simulink library "Computer_Library"  (Simulink 8.1)
settings: Solver=ode45  StartTime=0.0  StopTime=10.0  RelTol=1e-3
values from neighbouring files (symbols this model uses):
  A = 10    [CharTable.m]
  ARROW_DOWN = 48    [CharTable.m]
  ARROW_LEFT = 49    [CharTable.m]
  ARROW_RIGHT = 50    [CharTable.m]
  ARROW_UP = 47    [CharTable.m]
  ASTERISK = 39    [CharTable.m]
  B = 11    [CharTable.m]
  BACKSLASH = 43    [CharTable.m]
  C = 12    [CharTable.m]
  COLON = 40    [CharTable.m]
  COMMA = 53    [CharTable.m]
  CROSS = 38    [CharTable.m]
  CURSOR = 62    [CharTable.m]
  D = 13    [CharTable.m]
  DOT = 52    [CharTable.m]
  EQUAL = 44    [CharTable.m]
  EXCLAMATION_MARK = 55    [CharTable.m]
  F = 15    [CharTable.m]
  G = 16    [CharTable.m]
  GREATER_THAN = 46    [CharTable.m]
  H = 17    [CharTable.m]
  I = 18    [CharTable.m]
  J = 19    [CharTable.m]
  K = 20    [CharTable.m]
  L = 21    [CharTable.m]
  LEFT_PARENTHESES = 59    [CharTable.m]
  LESS_THAN = 45    [CharTable.m]
  M = 22    [CharTable.m]
  MINUS = 37    [CharTable.m]
  N = 23    [CharTable.m]
  O = 24    [CharTable.m]
  P = 25    [CharTable.m]
  PERCENT = 58    [CharTable.m]
  PLUS = 36    [CharTable.m]
  Q = 32    [CharTable.m]
  QUESTION_MARK = 54    [CharTable.m]
  QUOTE = 56    [CharTable.m]
  R = 26    [CharTable.m]
  RECTANGLE = 63    [CharTable.m]
  RIGHT_PARENTHESES = 60    [CharTable.m]
  RomCode = reshape(transpose(RomCode), [], 1)    [ROM.m]
  S = 27    [CharTable.m]
  SEMICOLON = 41    [CharTable.m]
  SHARP = 57    [CharTable.m]
  SLASH = 42    [CharTable.m]
  SPACE = 61    [CharTable.m]
  T = 28    [CharTable.m]
  U = 29    [CharTable.m]
  UNDERSCORE = 51    [CharTable.m]
  V = 30    [CharTable.m]
  W = 31    [CharTable.m]
  X = 33    [CharTable.m]
  Y = 34    [CharTable.m]
  Z = 35    [CharTable.m]
undefined symbols (not defined in the file or in its folder): char_0
libraries: Memory_Blocks_Lib x116, Byte_Multiplexers_Lib x44, commutil2 x18, Bit_Multiplexers_Lib x17, Decoders_Lib x9, simulink_extras x8, Logic_Operations_Lib x4, Byte_Demultiplexers_Lib x2, Arithmetic_Operations_Lib x2, dspsnks4 x1
(part 1 of 4)
settings Model: Creator=N  LastModifiedBy=uzivatel

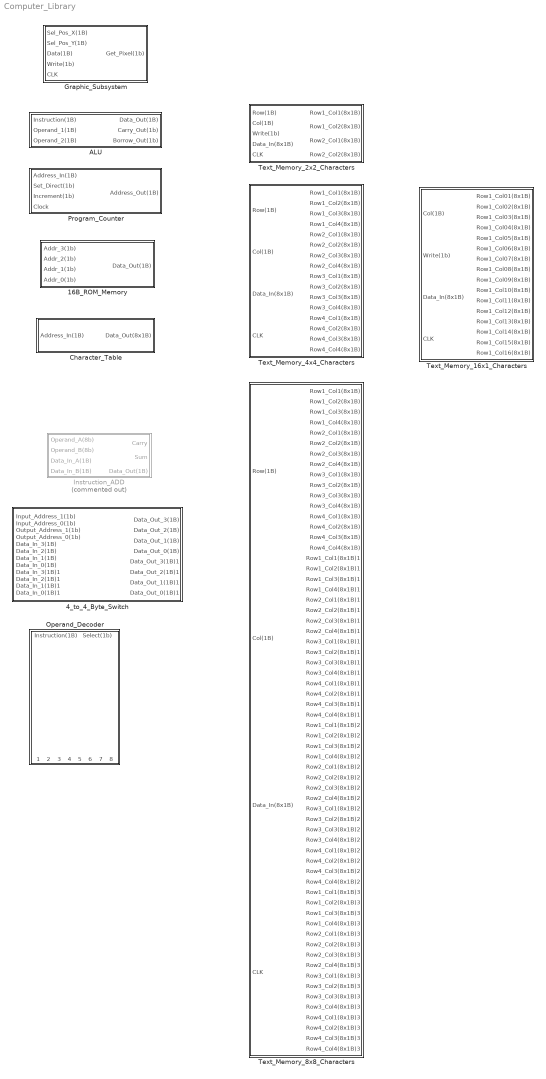
== system Computer_Library ==
  16B_ROM_Memory : Subsystem
  4_to_4_Byte_Switch : Subsystem
  ALU : Subsystem
  Character_Table : Subsystem
  Graphic_Subsystem : Subsystem
  Instruction_ADD : Subsystem  Commented=on
  Operand_Decoder : Subsystem
  Program_Counter : Subsystem
  Text_Memory_16x1_Characters : Subsystem
  Text_Memory_2x2_Characters : Subsystem
  Text_Memory_4x4_Characters : Subsystem
  Text_Memory_8x8_Characters : Subsystem

== system Computer_Library/16B_ROM_Memory ==
  Addr_3(1b) : Inport
  Addr_2(1b) : Inport  Port=2
  Addr_1(1b) : Inport  Port=3
  Addr_0(1b) : Inport  Port=4
  16_to_1_Byte_Multiplexer : Byte_Multiplexers_Lib/Byte_Multiplexers_Lib/Byte_Multiplexer_16_to_1
  Byte_00 : Constant  Value=RomCode(1)  OutDataTypeStr=uint8
  Byte_01 : Constant  Value=RomCode(2)  OutDataTypeStr=uint8
  Byte_02 : Constant  Value=RomCode(3)  OutDataTypeStr=uint8
  Byte_03 : Constant  Value=RomCode(4)  OutDataTypeStr=uint8
  Byte_04 : Constant  Value=RomCode(5)  OutDataTypeStr=uint8
  Byte_05 : Constant  Value=RomCode(6)  OutDataTypeStr=uint8
  Byte_06 : Constant  Value=RomCode(7)  OutDataTypeStr=uint8
  Byte_07 : Constant  Value=RomCode(8)  OutDataTypeStr=uint8
  Byte_08 : Constant  Value=RomCode(9)  OutDataTypeStr=uint8
  Byte_09 : Constant  Value=RomCode(10)  OutDataTypeStr=uint8
  Byte_10 : Constant  Value=RomCode(11)  OutDataTypeStr=uint8
  Byte_11 : Constant  Value=RomCode(12)  OutDataTypeStr=uint8
  Byte_12 : Constant  Value=RomCode(13)  OutDataTypeStr=uint8
  Byte_13 : Constant  Value=RomCode(14)  OutDataTypeStr=uint8
  Byte_14 : Constant  Value=RomCode(15)  OutDataTypeStr=uint8
  Byte_15 : Constant  Value=RomCode(16)  OutDataTypeStr=uint8
  Data_Out(1B) : Outport
  wires:
  16_to_1_Byte_Multiplexer/1 -> Data_Out(1B)/1
  Byte_00/1 -> 16_to_1_Byte_Multiplexer/20
  Byte_01/1 -> 16_to_1_Byte_Multiplexer/19
  Byte_02/1 -> 16_to_1_Byte_Multiplexer/18
  Byte_03/1 -> 16_to_1_Byte_Multiplexer/17
  Byte_04/1 -> 16_to_1_Byte_Multiplexer/16
  Byte_05/1 -> 16_to_1_Byte_Multiplexer/15
  Byte_06/1 -> 16_to_1_Byte_Multiplexer/14
  Byte_07/1 -> 16_to_1_Byte_Multiplexer/13
  Byte_08/1 -> 16_to_1_Byte_Multiplexer/12
  Byte_09/1 -> 16_to_1_Byte_Multiplexer/11
  Byte_10/1 -> 16_to_1_Byte_Multiplexer/10
  Byte_11/1 -> 16_to_1_Byte_Multiplexer/9
  Byte_12/1 -> 16_to_1_Byte_Multiplexer/8
  Byte_13/1 -> 16_to_1_Byte_Multiplexer/7
  Byte_14/1 -> 16_to_1_Byte_Multiplexer/6
  Byte_15/1 -> 16_to_1_Byte_Multiplexer/5
  Addr_3(1b)/1 -> 16_to_1_Byte_Multiplexer/1
  Addr_2(1b)/1 -> 16_to_1_Byte_Multiplexer/2
  Addr_1(1b)/1 -> 16_to_1_Byte_Multiplexer/3
  Addr_0(1b)/1 -> 16_to_1_Byte_Multiplexer/4

== system Computer_Library/4_to_4_Byte_Switch ==
  Input_Address_1(1b) : Inport
  Input_Address_0(1b) : Inport  Port=2
  Output_Address_1(1b) : Inport  Port=3
  Output_Address_0(1b) : Inport  Port=4
  Data_In_3(1B) : Inport  Port=5
  Data_In_2(1B) : Inport  Port=6
  Data_In_1(1B) : Inport  Port=7
  Data_In_0(1B) : Inport  Port=8
  Data_In_3(1B)1 : Inport  Port=9
  Data_In_2(1B)1 : Inport  Port=10
  Data_In_1(1B)1 : Inport  Port=11
  Data_In_0(1B)1 : Inport  Port=12
  1_to_4_Byte_Demultiplexer : Byte_Demultiplexers_Lib/Byte_Demultiplexers_Lib/Byte_Demultiplexer_1_to_4
  1_to_4_Byte_Demultiplexer1 : Byte_Demultiplexers_Lib/Byte_Demultiplexers_Lib/Byte_Demultiplexer_1_to_4
  4_to_1_Byte_Multiplexer1 : Byte_Multiplexers_Lib/Byte_Multiplexers_Lib/Byte_Multiplexer_4_to_1
  4_to_1_Byte_Multiplexer4 : Byte_Multiplexers_Lib/Byte_Multiplexers_Lib/Byte_Multiplexer_4_to_1
  Data_Out_3(1B) : Outport
  Data_Out_2(1B) : Outport  Port=2
  Data_Out_1(1B) : Outport  Port=3
  Data_Out_0(1B) : Outport  Port=4
  Data_Out_3(1B)1 : Outport  Port=5
  Data_Out_2(1B)1 : Outport  Port=6
  Data_Out_1(1B)1 : Outport  Port=7
  Data_Out_0(1B)1 : Outport  Port=8
  wires:
  4_to_1_Byte_Multiplexer4/1 -> 1_to_4_Byte_Demultiplexer/3
  1_to_4_Byte_Demultiplexer/1 -> Data_Out_3(1B)/1
  1_to_4_Byte_Demultiplexer/2 -> Data_Out_2(1B)/1
  1_to_4_Byte_Demultiplexer/3 -> Data_Out_1(1B)/1
  1_to_4_Byte_Demultiplexer/4 -> Data_Out_0(1B)/1
  Data_In_0(1B)/1 -> 4_to_1_Byte_Multiplexer4/6
  Data_In_1(1B)/1 -> 4_to_1_Byte_Multiplexer4/5
  Data_In_2(1B)/1 -> 4_to_1_Byte_Multiplexer4/4
  Data_In_3(1B)/1 -> 4_to_1_Byte_Multiplexer4/3
  Input_Address_0(1b)/1 -> 1_to_4_Byte_Demultiplexer1/2, 4_to_1_Byte_Multiplexer4/2
  Input_Address_1(1b)/1 -> 1_to_4_Byte_Demultiplexer1/1, 4_to_1_Byte_Multiplexer4/1
  Output_Address_0(1b)/1 -> 4_to_1_Byte_Multiplexer1/2, 1_to_4_Byte_Demultiplexer/2
  Output_Address_1(1b)/1 -> 4_to_1_Byte_Multiplexer1/1, 1_to_4_Byte_Demultiplexer/1
  4_to_1_Byte_Multiplexer1/1 -> 1_to_4_Byte_Demultiplexer1/3
  1_to_4_Byte_Demultiplexer1/1 -> Data_Out_3(1B)1/1
  1_to_4_Byte_Demultiplexer1/2 -> Data_Out_2(1B)1/1
  1_to_4_Byte_Demultiplexer1/3 -> Data_Out_1(1B)1/1
  1_to_4_Byte_Demultiplexer1/4 -> Data_Out_0(1B)1/1
  Data_In_0(1B)1/1 -> 4_to_1_Byte_Multiplexer1/6
  Data_In_1(1B)1/1 -> 4_to_1_Byte_Multiplexer1/5
  Data_In_2(1B)1/1 -> 4_to_1_Byte_Multiplexer1/4
  Data_In_3(1B)1/1 -> 4_to_1_Byte_Multiplexer1/3

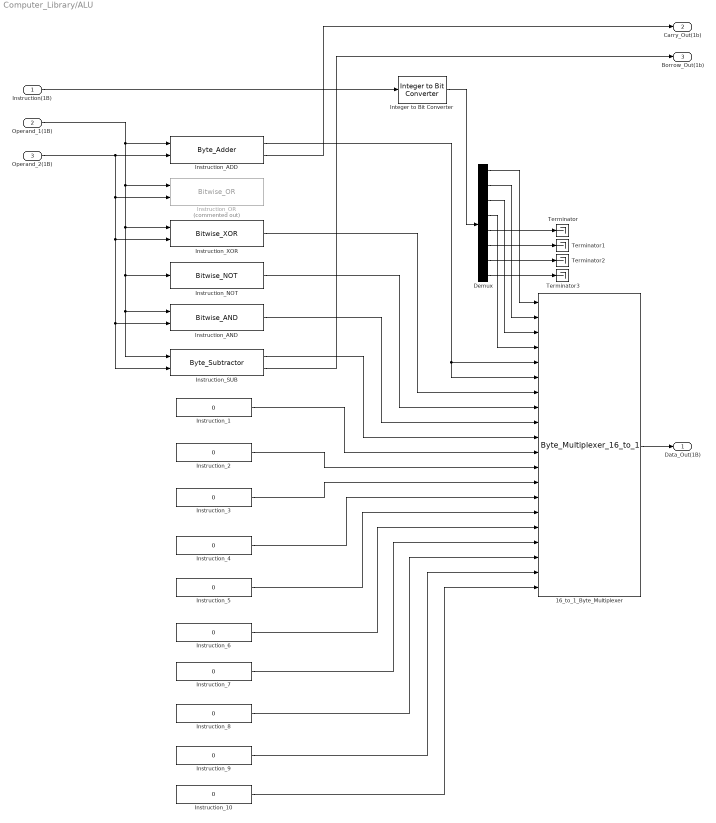
== system Computer_Library/ALU ==
  Instruction(1B) : Inport
  Operand_1(1B) : Inport  Port=2
  Operand_2(1B) : Inport  Port=3
  16_to_1_Byte_Multiplexer : Byte_Multiplexers_Lib/Byte_Multiplexers_Lib/Byte_Multiplexer_16_to_1
  Demux : Demux  Outputs=8
  Instruction_{1..10} (10 alike) : Constant  Value=0  OutDataTypeStr=uint8
  Instruction_ADD : Arithmetic_Operations_Lib/Arithmetic_Operations_Lib/Byte_Adder
  Instruction_AND : Logic_Operations_Lib/Logic_Operations_Lib/Bitwise_AND
  Instruction_NOT : Logic_Operations_Lib/Logic_Operations_Lib/Bitwise_NOT
  Instruction_OR : Logic_Operations_Lib/Logic_Operations_Lib/Bitwise_OR  Commented=on
  Instruction_SUB : Arithmetic_Operations_Lib/Arithmetic_Operations_Lib/Byte_Subtractor
  Instruction_XOR : Logic_Operations_Lib/Logic_Operations_Lib/Bitwise_XOR
  Integer to Bit Converter : commutil2/Integer to Bit Converter  nbits=8  signedInputValues=Unsigned  bitOrder=MSB first  outDtype=boolean
  Terminator{,1..3} (4 alike) : Terminator
  Data_Out(1B) : Outport
  Carry_Out(1b) : Outport  Port=2
  Borrow_Out(1b) : Outport  Port=3
  wires:
  Operand_1(1B)/1 -> Instruction_OR/1, Instruction_AND/1, Instruction_SUB/1, Instruction_NOT/1, Instruction_XOR/1, Instruction_ADD/1
  Operand_2(1B)/1 -> Instruction_OR/2, Instruction_AND/2, Instruction_SUB/2, Instruction_XOR/2, Instruction_ADD/2
  Instruction_ADD/1 -> 16_to_1_Byte_Multiplexer/6, 16_to_1_Byte_Multiplexer/5
  Instruction_XOR/1 -> 16_to_1_Byte_Multiplexer/7
  Instruction_NOT/1 -> 16_to_1_Byte_Multiplexer/8
  Instruction_AND/1 -> 16_to_1_Byte_Multiplexer/9
  Instruction_SUB/1 -> 16_to_1_Byte_Multiplexer/10
  Instruction_1/1 -> 16_to_1_Byte_Multiplexer/11
  Instruction_2/1 -> 16_to_1_Byte_Multiplexer/12
  Instruction_3/1 -> 16_to_1_Byte_Multiplexer/13
  Instruction_4/1 -> 16_to_1_Byte_Multiplexer/14
  Instruction_5/1 -> 16_to_1_Byte_Multiplexer/15
  Instruction_6/1 -> 16_to_1_Byte_Multiplexer/16
  Instruction_7/1 -> 16_to_1_Byte_Multiplexer/17
  Instruction_8/1 -> 16_to_1_Byte_Multiplexer/18
  Instruction_9/1 -> 16_to_1_Byte_Multiplexer/19
  Instruction_10/1 -> 16_to_1_Byte_Multiplexer/20
  Instruction(1B)/1 -> Integer to Bit Converter/1
  16_to_1_Byte_Multiplexer/1 -> Data_Out(1B)/1
  Integer to Bit Converter/1 -> Demux/1
  Demux/4 -> 16_to_1_Byte_Multiplexer/4
  Demux/3 -> 16_to_1_Byte_Multiplexer/3
  Demux/2 -> 16_to_1_Byte_Multiplexer/2
  Demux/1 -> 16_to_1_Byte_Multiplexer/1
  Demux/8 -> Terminator3/1
  Demux/7 -> Terminator2/1
  Demux/6 -> Terminator1/1
  Demux/5 -> Terminator/1
  Instruction_ADD/2 -> Carry_Out(1b)/1
  Instruction_SUB/2 -> Borrow_Out(1b)/1

== system Computer_Library/Character_Table ==
  note: Toto nie su stlpce ale riadky, treba opravit!!!
  Address_In(1B) : Inport
  4_to_1_Byte_Multiplexer{,1..7} (8 alike) : Byte_Multiplexers_Lib/Byte_Multiplexers_Lib/Byte_Multiplexer_4_to_1
  Characters(0..F) : Subsystem
  Characters(ARROW_DOWN..RECTANGLE) : Subsystem
  Characters(G..W) : Subsystem
  Characters(Q..ARROW_UP) : Subsystem
  Demux : Demux  Outputs=8
  Integer to Bit Converter : commutil2/Integer to Bit Converter  nbits=8  signedInputValues=Unsigned  bitOrder=MSB first  outDtype=uint8
  Mux : Mux  Inputs=8
  Terminator : Terminator
  Terminator1 : Terminator
  Data_Out(8x1B) : Outport
  wires:
  Characters(0..F)/3(Column_3(1B)) -> 4_to_1_Byte_Multiplexer2/6
  Characters(Q..ARROW_UP)/6(Column_6(1B)) -> 4_to_1_Byte_Multiplexer5/4
  Characters(Q..ARROW_UP)/7(Column_7(1B)) -> 4_to_1_Byte_Multiplexer6/4
  Characters(ARROW_DOWN..RECTANGLE)/2(Column_2(1B)) -> 4_to_1_Byte_Multiplexer1/3
  Characters(0..F)/2(Column_2(1B)) -> 4_to_1_Byte_Multiplexer1/6
  Characters(Q..ARROW_UP)/2(Column_2(1B)) -> 4_to_1_Byte_Multiplexer1/4
  Characters(ARROW_DOWN..RECTANGLE)/7(Column_7(1B)) -> 4_to_1_Byte_Multiplexer6/3
  Characters(G..W)/2(Column_2(1B)) -> 4_to_1_Byte_Multiplexer1/5
  Characters(ARROW_DOWN..RECTANGLE)/8(Column_8(1B)) -> 4_to_1_Byte_Multiplexer7/3
  Characters(G..W)/4(Column_4(1B)) -> 4_to_1_Byte_Multiplexer3/5
  Characters(ARROW_DOWN..RECTANGLE)/6(Column_6(1B)) -> 4_to_1_Byte_Multiplexer5/3
  Characters(G..W)/3(Column_3(1B)) -> 4_to_1_Byte_Multiplexer2/5
  Characters(Q..ARROW_UP)/5(Column_5(1B)) -> 4_to_1_Byte_Multiplexer4/4
  Characters(0..F)/4(Column_4(1B)) -> 4_to_1_Byte_Multiplexer3/6
  Characters(Q..ARROW_UP)/1(Column_1(1B)) -> 4_to_1_Byte_Multiplexer/4
  Characters(ARROW_DOWN..RECTANGLE)/3(Column_3(1B)) -> 4_to_1_Byte_Multiplexer2/3
  Characters(Q..ARROW_UP)/3(Column_3(1B)) -> 4_to_1_Byte_Multiplexer2/4
  Characters(G..W)/6(Column_6(1B)) -> 4_to_1_Byte_Multiplexer5/5
  Characters(0..F)/7(Column_7(1B)) -> 4_to_1_Byte_Multiplexer6/6
  Characters(G..W)/7(Column_7(1B)) -> 4_to_1_Byte_Multiplexer6/5
  Characters(0..F)/8(Column_8(1B)) -> 4_to_1_Byte_Multiplexer7/6
  Characters(Q..ARROW_UP)/8(Column_8(1B)) -> 4_to_1_Byte_Multiplexer7/4
  Characters(ARROW_DOWN..RECTANGLE)/5(Column_5(1B)) -> 4_to_1_Byte_Multiplexer4/3
  Characters(G..W)/8(Column_8(1B)) -> 4_to_1_Byte_Multiplexer7/5
  Demux/3 -> 4_to_1_Byte_Multiplexer1/1, 4_to_1_Byte_Multiplexer2/1, 4_to_1_Byte_Multiplexer4/1, 4_to_1_Byte_Multiplexer5/1, 4_to_1_Byte_Multiplexer6/1, 4_to_1_Byte_Multiplexer7/1, 4_to_1_Byte_Multiplexer3/1, 4_to_1_Byte_Multiplexer/1
  Characters(Q..ARROW_UP)/4(Column_4(1B)) -> 4_to_1_Byte_Multiplexer3/4
  Demux/4 -> 4_to_1_Byte_Multiplexer1/2, 4_to_1_Byte_Multiplexer2/2, 4_to_1_Byte_Multiplexer3/2, 4_to_1_Byte_Multiplexer4/2, 4_to_1_Byte_Multiplexer5/2, 4_to_1_Byte_Multiplexer6/2, 4_to_1_Byte_Multiplexer7/2, 4_to_1_Byte_Multiplexer/2
  Characters(0..F)/1(Column_1(1B)) -> 4_to_1_Byte_Multiplexer/6
  Characters(G..W)/1(Column_1(1B)) -> 4_to_1_Byte_Multiplexer/5
  Characters(0..F)/5(Column_5(1B)) -> 4_to_1_Byte_Multiplexer4/6
  Characters(G..W)/5(Column_5(1B)) -> 4_to_1_Byte_Multiplexer4/5
  Characters(0..F)/6(Column_6(1B)) -> 4_to_1_Byte_Multiplexer5/6
  Characters(ARROW_DOWN..RECTANGLE)/1(Column_1(1B)) -> 4_to_1_Byte_Multiplexer/3
  Characters(ARROW_DOWN..RECTANGLE)/4(Column_4(1B)) -> 4_to_1_Byte_Multiplexer3/3
  Demux/8 -> Characters(ARROW_DOWN..RECTANGLE)/4(Address_0_In(1b)), Characters(Q..ARROW_UP)/4(Address_0_In(1b)), Characters(G..W)/4(Address_0_In(1b)), Characters(0..F)/4(Address_0_In(1b))
  Demux/6 -> Characters(ARROW_DOWN..RECTANGLE)/2(Address_2_In(1b)), Characters(Q..ARROW_UP)/2(Address_2_In(1b)), Characters(0..F)/2(Address_2_In(1b)), Characters(G..W)/2(Address_2_In(1b))
  4_to_1_Byte_Multiplexer6/1 -> Mux/7
  Demux/5 -> Characters(ARROW_DOWN..RECTANGLE)/1(Address_3_In(1b)), Characters(Q..ARROW_UP)/1(Address_3_In(1b)), Characters(G..W)/1(Address_3_In(1b)), Characters(0..F)/1(Address_3_In(1b))
  4_to_1_Byte_Multiplexer1/1 -> Mux/2
  4_to_1_Byte_Multiplexer5/1 -> Mux/6
  4_to_1_Byte_Multiplexer2/1 -> Mux/3
  4_to_1_Byte_Multiplexer3/1 -> Mux/4
  4_to_1_Byte_Multiplexer7/1 -> Mux/8
  4_to_1_Byte_Multiplexer/1 -> Mux/1
  Demux/7 -> Characters(ARROW_DOWN..RECTANGLE)/3(Address_1_In(1b)), Characters(Q..ARROW_UP)/3(Address_1_In(1b)), Characters(0..F)/3(Address_1_In(1b)), Characters(G..W)/3(Address_1_In(1b))
  4_to_1_Byte_Multiplexer4/1 -> Mux/5
  Address_In(1B)/1 -> Integer to Bit Converter/1
  Demux/1 -> Terminator/1
  Demux/2 -> Terminator1/1
  Integer to Bit Converter/1 -> Demux/1
  Mux/1 -> Data_Out(8x1B)/1

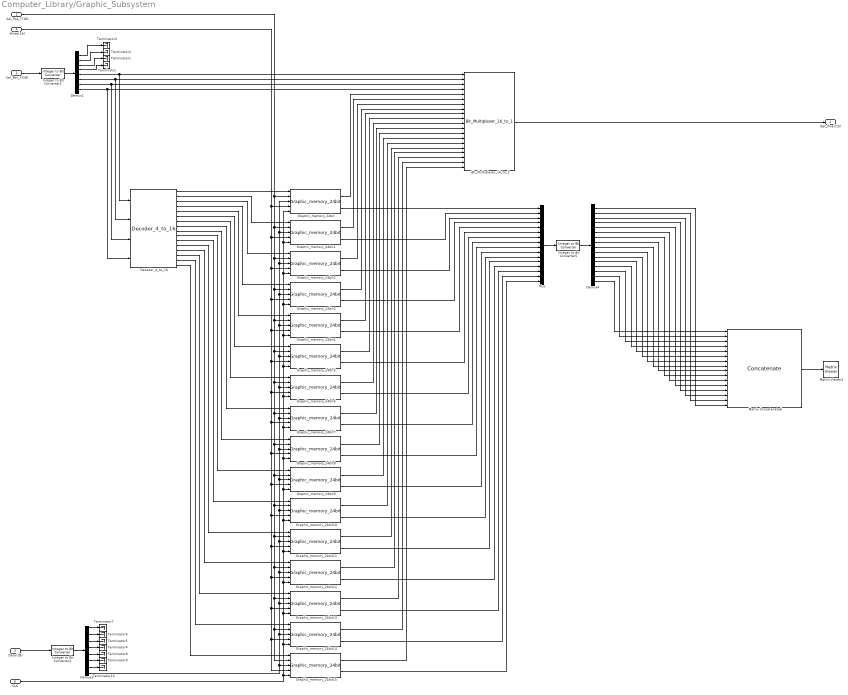
== system Computer_Library/Graphic_Subsystem ==
  Sel_Pos_X(1B) : Inport
  Sel_Pos_Y(1B) : Inport  Port=2
  Data(1B) : Inport  Port=3
  Write(1b) : Inport  Port=4
  CLK : Inport  Port=5
  Bit_Multiplexer_16_to_1 : Bit_Multiplexers_Lib/Bit_Multiplexers_Lib/Bit_Multiplexer_16_to_1
  Decoder_4_to_16 : Decoders_Lib/Decoders_Lib/Decoder_4_to_16
  Demux1 : Demux  Outputs=8
  Demux2 : Demux  Outputs=8
  Demux4 : Demux  Outputs=16
  Graphic_memory_24bit{,1..15} (16 alike) : Memory_Blocks_Lib/Memory_Blocks_Lib/Graphic_memory_24bit
  Integer to Bit Converter1 : commutil2/Integer to Bit Converter  nbits=8  signedInputValues=Unsigned  bitOrder=MSB first  outDtype=boolean
  Integer to Bit Converter2 : commutil2/Integer to Bit Converter  nbits=8  signedInputValues=Unsigned  bitOrder=MSB first  outDtype=boolean
  Integer to Bit Converter5 : commutil2/Integer to Bit Converter  nbits=24  signedInputValues=Unsigned  bitOrder=LSB first  outDtype=uint32
  Matrix Concatenate6 : Concatenate  NumInputs=16  Mode=Multidimensional array  ConcatenateDimension=2
  Matrix Viewer2 : dspsnks4/Matrix Viewer  ImageParams=off  CMapStr=[0 0.3 0; 0 1 0]  AxisColorbar=on  AxisParams=off  AxisOrigin=Upper left corner  XLabel=X-axis  YLabel=Y-axis  ZLabel=Z-axis  FigPos=[1700 500 200 350]  AxisZoom=on
      settings: YMin=0  YMax=1
  Mux : Mux  Inputs=16
  Terminator{,1..10} (11 alike) : Terminator
  Get_Pixel(1b) : Outport
  wires:
  Sel_Pos_Y(1B)/1 -> Graphic_memory_24bit/2, Graphic_memory_24bit1/2, Graphic_memory_24bit2/2, Graphic_memory_24bit3/2, Graphic_memory_24bit4/2, Graphic_memory_24bit5/2, Graphic_memory_24bit6/2, Graphic_memory_24bit7/2, Graphic_memory_24bit8/2, Graphic_memory_24bit9/2, Graphic_memory_24bit10/2, Graphic_memory_24bit11/2, Graphic_memory_24bit12/2, Graphic_memory_24bit13/2, Graphic_memory_24bit14/2, Graphic_memory_24bit15/2
  Demux1/1 -> Terminator3/1
  Demux1/2 -> Terminator2/1
  Demux1/5 -> Decoder_4_to_16/1, Bit_Multiplexer_16_to_1/1
  Demux1/7 -> Bit_Multiplexer_16_to_1/3, Decoder_4_to_16/3
  Sel_Pos_X(1B)/1 -> Integer to Bit Converter1/1
  Demux2/8 -> Graphic_memory_24bit15/3, Graphic_memory_24bit14/3, Graphic_memory_24bit13/3, Graphic_memory_24bit12/3, Graphic_memory_24bit11/3, Graphic_memory_24bit10/3, Graphic_memory_24bit9/3, Graphic_memory_24bit8/3, Graphic_memory_24bit7/3, Graphic_memory_24bit6/3, Graphic_memory_24bit5/3, Graphic_memory_24bit4/3, Graphic_memory_24bit3/3, Graphic_memory_24bit2/3, Graphic_memory_24bit1/3, Graphic_memory_24bit/3
  Demux1/6 -> Bit_Multiplexer_16_to_1/2, Decoder_4_to_16/2
  Demux1/8 -> Bit_Multiplexer_16_to_1/4, Decoder_4_to_16/4
  Integer to Bit Converter1/1 -> Demux1/1
  Demux1/4 -> Terminator/1
  Demux1/3 -> Terminator1/1
  Mux/1 -> Integer to Bit Converter5/1
  Decoder_4_to_16/13 -> Graphic_memory_24bit12/1
  Matrix Concatenate6/1 -> Matrix Viewer2/1
  Integer to Bit Converter5/1 -> Demux4/1
  Graphic_memory_24bit2/2 -> Mux/3
  Decoder_4_to_16/6 -> Graphic_memory_24bit5/1
  Graphic_memory_24bit9/2 -> Mux/10
  Decoder_4_to_16/11 -> Graphic_memory_24bit10/1
  Graphic_memory_24bit4/2 -> Mux/5
  Graphic_memory_24bit/2 -> Mux/1
  Graphic_memory_24bit13/2 -> Mux/14
  Decoder_4_to_16/3 -> Graphic_memory_24bit2/1
  Graphic_memory_24bit15/2 -> Mux/16
  Decoder_4_to_16/16 -> Graphic_memory_24bit15/1
  CLK/1 -> Graphic_memory_24bit15/5, Graphic_memory_24bit14/5, Graphic_memory_24bit13/5, Graphic_memory_24bit12/5, Graphic_memory_24bit11/5, Graphic_memory_24bit10/5, Graphic_memory_24bit9/5, Graphic_memory_24bit8/5, Graphic_memory_24bit7/5, Graphic_memory_24bit6/5, Graphic_memory_24bit5/5, Graphic_memory_24bit4/5, Graphic_memory_24bit3/5, Graphic_memory_24bit2/5, Graphic_memory_24bit/5, Graphic_memory_24bit1/5
  Decoder_4_to_16/1 -> Graphic_memory_24bit/1
  Graphic_memory_24bit3/2 -> Mux/4
  Decoder_4_to_16/10 -> Graphic_memory_24bit9/1
  Graphic_memory_24bit12/2 -> Mux/13
  Decoder_4_to_16/12 -> Graphic_memory_24bit11/1
  Graphic_memory_24bit5/2 -> Mux/6
  Graphic_memory_24bit1/2 -> Mux/2
  Decoder_4_to_16/2 -> Graphic_memory_24bit1/1
  Decoder_4_to_16/4 -> Graphic_memory_24bit3/1
  Decoder_4_to_16/9 -> Graphic_memory_24bit8/1
  Graphic_memory_24bit11/2 -> Mux/12
  Decoder_4_to_16/5 -> Graphic_memory_24bit4/1
  Graphic_memory_24bit6/2 -> Mux/7
  Graphic_memory_24bit7/2 -> Mux/8
  Graphic_memory_24bit8/2 -> Mux/9
  Decoder_4_to_16/14 -> Graphic_memory_24bit13/1
  Graphic_memory_24bit14/2 -> Mux/15
  Decoder_4_to_16/15 -> Graphic_memory_24bit14/1
  Decoder_4_to_16/8 -> Graphic_memory_24bit7/1
  Decoder_4_to_16/7 -> Graphic_memory_24bit6/1
  Graphic_memory_24bit10/2 -> Mux/11
  Demux4/16 -> Matrix Concatenate6/1
  Demux4/15 -> Matrix Concatenate6/2
  Demux4/14 -> Matrix Concatenate6/3
  Demux4/13 -> Matrix Concatenate6/4
  Demux4/12 -> Matrix Concatenate6/5
  Demux4/11 -> Matrix Concatenate6/6
  Demux4/10 -> Matrix Concatenate6/7
  Demux4/9 -> Matrix Concatenate6/8
  Demux4/8 -> Matrix Concatenate6/9
  Demux4/7 -> Matrix Concatenate6/10
  Demux4/6 -> Matrix Concatenate6/11
  Demux4/5 -> Matrix Concatenate6/12
  Demux4/4 -> Matrix Concatenate6/13
  Demux4/3 -> Matrix Concatenate6/14
  Demux4/2 -> Matrix Concatenate6/15
  Demux4/1 -> Matrix Concatenate6/16
  Write(1b)/1 -> Graphic_memory_24bit/4, Graphic_memory_24bit1/4, Graphic_memory_24bit2/4, Graphic_memory_24bit3/4, Graphic_memory_24bit4/4, Graphic_memory_24bit5/4, Graphic_memory_24bit6/4, Graphic_memory_24bit7/4, Graphic_memory_24bit8/4, Graphic_memory_24bit9/4, Graphic_memory_24bit10/4, Graphic_memory_24bit11/4, Graphic_memory_24bit12/4, Graphic_memory_24bit13/4, Graphic_memory_24bit14/4, Graphic_memory_24bit15/4
  Demux2/1 -> Terminator7/1
  Demux2/2 -> Terminator6/1
  Integer to Bit Converter2/1 -> Demux2/1
  Demux2/4 -> Terminator4/1
  Demux2/3 -> Terminator5/1
  Data(1B)/1 -> Integer to Bit Converter2/1
  Demux2/7 -> Terminator10/1
  Demux2/6 -> Terminator9/1
  Demux2/5 -> Terminator8/1
  Graphic_memory_24bit/1 -> Bit_Multiplexer_16_to_1/5
  Graphic_memory_24bit1/1 -> Bit_Multiplexer_16_to_1/6
  Graphic_memory_24bit2/1 -> Bit_Multiplexer_16_to_1/7
  Graphic_memory_24bit3/1 -> Bit_Multiplexer_16_to_1/8
  Graphic_memory_24bit4/1 -> Bit_Multiplexer_16_to_1/9
  Graphic_memory_24bit5/1 -> Bit_Multiplexer_16_to_1/10
  Graphic_memory_24bit6/1 -> Bit_Multiplexer_16_to_1/11
  Graphic_memory_24bit7/1 -> Bit_Multiplexer_16_to_1/12
  Graphic_memory_24bit8/1 -> Bit_Multiplexer_16_to_1/13
  Graphic_memory_24bit9/1 -> Bit_Multiplexer_16_to_1/14
  Graphic_memory_24bit10/1 -> Bit_Multiplexer_16_to_1/15
  Graphic_memory_24bit11/1 -> Bit_Multiplexer_16_to_1/16
  Graphic_memory_24bit12/1 -> Bit_Multiplexer_16_to_1/17
  Graphic_memory_24bit13/1 -> Bit_Multiplexer_16_to_1/18
  Graphic_memory_24bit14/1 -> Bit_Multiplexer_16_to_1/19
  Graphic_memory_24bit15/1 -> Bit_Multiplexer_16_to_1/20
  Bit_Multiplexer_16_to_1/1 -> Get_Pixel(1b)/1

== system Computer_Library/Instruction_ADD ==
  Operand_A(8b) : Inport
  Operand_B(8b) : Inport  Port=2
  Data_In_A(1B) : Inport  Port=3
  Data_In_B(1B) : Inport  Port=4
  Bit to Integer Converter1 : commutil2/Bit to Integer Converter  nbits=8  bitOrder=MSB first  signedOutputValues=Unsigned  outDtype=uint8  outDtypeSigned=Inherit via internal rule
  Constant : Constant  Value=0
  Demux1 : Demux  Outputs=8
  Demux17 : Demux  Outputs=8
  Full_Adder : Subsystem
  Full_Adder1 : Subsystem
  Full_Adder2 : Subsystem
  Full_Adder3 : Subsystem
  Full_Adder4 : Subsystem
  Full_Adder5 : Subsystem
  Full_Adder6 : Subsystem
  Full_Adder7 : Subsystem
  Integer to Bit Converter : commutil2/Integer to Bit Converter  nbits=8  signedInputValues=Unsigned  bitOrder=MSB first  outDtype=boolean
  Integer to Bit Converter1 : commutil2/Integer to Bit Converter  nbits=8  signedInputValues=Unsigned  bitOrder=MSB first  outDtype=boolean
  Mux : Mux  Inputs=8
  Carry : Outport
  Sum : Outport  Port=2
  Data_Out(1B) : Outport  Port=3
  wires:
  Demux17/4 -> Full_Adder3/1(A)
  Operand_A(8b)/1 -> Demux17/1
  Demux17/8 -> Full_Adder7/1(A)
  Demux1/8 -> Full_Adder7/2(B)
  Full_Adder/2(Sum) -> Mux/1
  Full_Adder7/2(Sum) -> Mux/8
  Full_Adder6/2(Sum) -> Mux/7
  Full_Adder5/2(Sum) -> Mux/6
  Full_Adder4/2(Sum) -> Mux/5
  Full_Adder3/1(Carry_Out) -> Full_Adder2/3(Carry_In)
  Full_Adder3/2(Sum) -> Mux/4
  Full_Adder2/2(Sum) -> Mux/3
  Full_Adder1/2(Sum) -> Mux/2
  Operand_B(8b)/1 -> Demux1/1
  Full_Adder7/1(Carry_Out) -> Full_Adder6/3(Carry_In)
  Full_Adder6/1(Carry_Out) -> Full_Adder5/3(Carry_In)
  Full_Adder5/1(Carry_Out) -> Full_Adder4/3(Carry_In)
  Full_Adder4/1(Carry_Out) -> Full_Adder3/3(Carry_In)
  Full_Adder2/1(Carry_Out) -> Full_Adder1/3(Carry_In)
  Full_Adder1/1(Carry_Out) -> Full_Adder/3(Carry_In)
  Full_Adder/1(Carry_Out) -> Carry/1
  Mux/1 -> Sum/1
  Demux1/7 -> Full_Adder6/2(B)
  Demux17/7 -> Full_Adder6/1(A)
  Demux1/6 -> Full_Adder5/2(B)
  Demux17/6 -> Full_Adder5/1(A)
  Demux1/5 -> Full_Adder4/2(B)
  Demux17/5 -> Full_Adder4/1(A)
  Demux1/4 -> Full_Adder3/2(B)
  Demux17/3 -> Full_Adder2/1(A)
  Demux1/3 -> Full_Adder2/2(B)
  Demux1/2 -> Full_Adder1/2(B)
  Demux17/2 -> Full_Adder1/1(A)
  Demux1/1 -> Full_Adder/2(B)
  Demux17/1 -> Full_Adder/1(A)
  Constant/1 -> Full_Adder7/3(Carry_In)
  Data_In_A(1B)/1 -> Integer to Bit Converter/1
  Data_In_B(1B)/1 -> Integer to Bit Converter1/1
  Bit to Integer Converter1/1 -> Data_Out(1B)/1

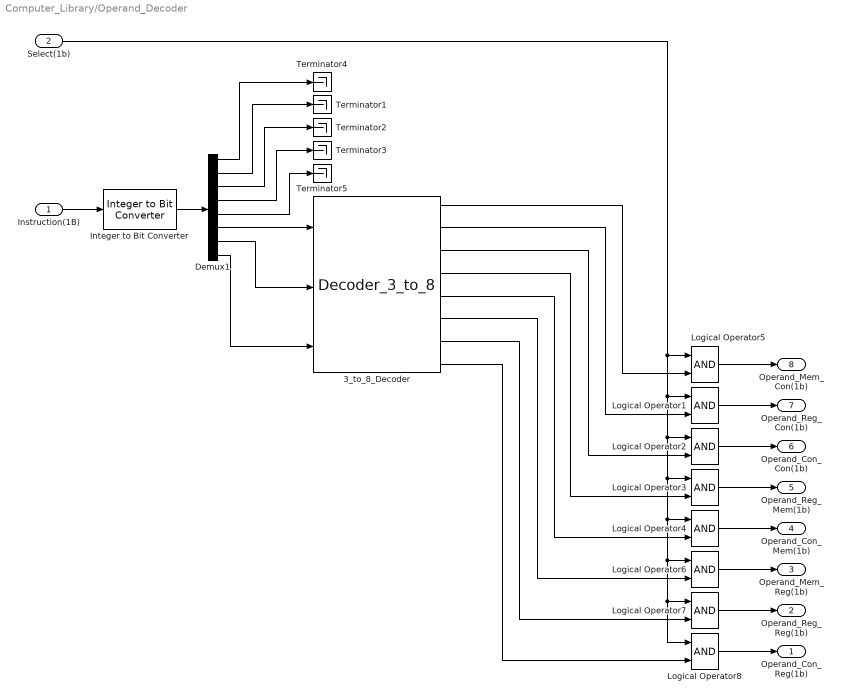
== system Computer_Library/Operand_Decoder ==
  Instruction(1B) : Inport
  Select(1b) : Inport  Port=2
  3_to_8_Decoder : Decoders_Lib/Decoders_Lib/Decoder_3_to_8
  Demux1 : Demux  Outputs=8
  Integer to Bit Converter : commutil2/Integer to Bit Converter  nbits=8  signedInputValues=Unsigned  bitOrder=MSB first  outDtype=boolean
  Logical Operator{1..8} (8 alike) : Logic  IconShape=distinctive  AllPortsSameDT=off  OutDataTypeStr=boolean
  Terminator{1..5} (5 alike) : Terminator
  Operand_Con_Reg(1b) : Outport
  Operand_Reg_Reg(1b) : Outport  Port=2
  Operand_Mem_Reg(1b) : Outport  Port=3
  Operand_Con_Mem(1b) : Outport  Port=4
  Operand_Reg_Mem(1b) : Outport  Port=5
  Operand_Con_Con(1b) : Outport  Port=6
  Operand_Reg_Con(1b) : Outport  Port=7
  Operand_Mem_Con(1b) : Outport  Port=8
  wires:
  Demux1/8 -> 3_to_8_Decoder/3
  Demux1/7 -> 3_to_8_Decoder/2
  Demux1/6 -> 3_to_8_Decoder/1
  3_to_8_Decoder/8 -> Logical Operator8/2
  3_to_8_Decoder/2 -> Logical Operator1/2
  3_to_8_Decoder/7 -> Logical Operator7/2
  3_to_8_Decoder/5 -> Logical Operator4/2
  3_to_8_Decoder/4 -> Logical Operator3/2
  3_to_8_Decoder/6 -> Logical Operator6/2
  3_to_8_Decoder/1 -> Logical Operator5/2
  3_to_8_Decoder/3 -> Logical Operator2/2
  Instruction(1B)/1 -> Integer to Bit Converter/1
  Integer to Bit Converter/1 -> Demux1/1
  Demux1/1 -> Terminator4/1
  Demux1/2 -> Terminator1/1
  Demux1/3 -> Terminator2/1
  Demux1/4 -> Terminator3/1
  Demux1/5 -> Terminator5/1
  Select(1b)/1 -> Logical Operator2/1, Logical Operator3/1, Logical Operator4/1, Logical Operator6/1, Logical Operator7/1, Logical Operator8/1, Logical Operator1/1, Logical Operator5/1
  Logical Operator5/1 -> Operand_Mem_Con(1b)/1
  Logical Operator1/1 -> Operand_Reg_Con(1b)/1
  Logical Operator2/1 -> Operand_Con_Con(1b)/1
  Logical Operator3/1 -> Operand_Reg_Mem(1b)/1
  Logical Operator4/1 -> Operand_Con_Mem(1b)/1
  Logical Operator6/1 -> Operand_Mem_Reg(1b)/1
  Logical Operator7/1 -> Operand_Reg_Reg(1b)/1
  Logical Operator8/1 -> Operand_Con_Reg(1b)/1

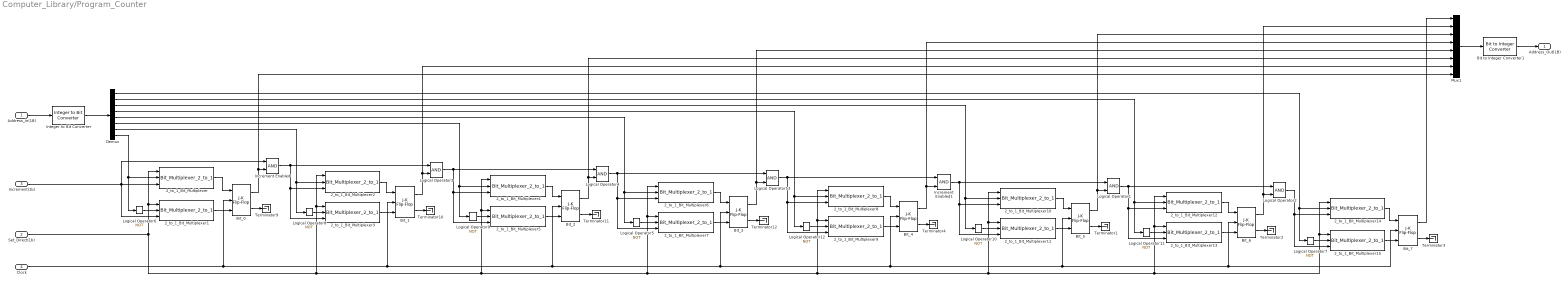
== system Computer_Library/Program_Counter ==
  Address_In(1B) : Inport
  Set_Direct(1b) : Inport  Port=2
  Increment(1b) : Inport  Port=3
  Clock : Inport  Port=4
  2_to_1_Bit_Multiplexer{,1..15} (16 alike) : Bit_Multiplexers_Lib/Bit_Multiplexers_Lib/Bit_Multiplexer_2_to_1
  Bit to Integer Converter1 : commutil2/Bit to Integer Converter  nbits=8  bitOrder=MSB first  signedOutputValues=Unsigned  outDtype=uint8  outDtypeSigned=Inherit via internal rule
  Bit_{0..7} (8 alike) : simulink_extras/Flip Flops/J-K Flip-Flop  initial_condition=0
  Demux : Demux  Outputs=8
  Increment Enabled : Logic  IconShape=distinctive  AllPortsSameDT=off  OutDataTypeStr=boolean
  Increment Enabled1 : Logic  IconShape=distinctive  AllPortsSameDT=off  OutDataTypeStr=boolean
  Integer to Bit Converter : commutil2/Integer to Bit Converter  nbits=8  signedInputValues=Unsigned  bitOrder=MSB first  outDtype=boolean
  Logical Operator{1..4,13} (5 alike) : Logic  IconShape=distinctive  AllPortsSameDT=off  OutDataTypeStr=boolean
  Logical Operator{5..12} (8 alike) : Logic  Operator=NOT  IconShape=distinctive  AllPortsSameDT=off  OutDataTypeStr=boolean
  Mux1 : Mux  Inputs=8
  Terminator{1..4,9..12} (8 alike) : Terminator
  Address_Out(1B) : Outport
  wires:
  Increment(1b)/1 -> 2_to_1_Bit_Multiplexer1/3, 2_to_1_Bit_Multiplexer/3, Increment Enabled/1
  Bit_0/2 -> Terminator9/1
  Bit_1/2 -> Terminator10/1
  Bit_2/2 -> Terminator11/1
  Increment Enabled/1 -> Logical Operator3/1, 2_to_1_Bit_Multiplexer3/3, 2_to_1_Bit_Multiplexer2/3
  Bit_1/1 -> Mux1/7, Logical Operator3/2
  Logical Operator3/1 -> 2_to_1_Bit_Multiplexer5/3, 2_to_1_Bit_Multiplexer4/3, Logical Operator4/1
  Bit_3/2 -> Terminator12/1
  Bit_2/1 -> Mux1/6, Logical Operator4/2
  Bit_3/1 -> Logical Operator13/2, Mux1/5
  Bit to Integer Converter1/1 -> Address_Out(1B)/1
  Mux1/1 -> Bit to Integer Converter1/1
  Address_In(1B)/1 -> Integer to Bit Converter/1
  Demux/8 -> Logical Operator6/1, 2_to_1_Bit_Multiplexer/2
  2_to_1_Bit_Multiplexer1/1 -> Bit_0/3
  2_to_1_Bit_Multiplexer/1 -> Bit_0/1
  Logical Operator6/1 -> 2_to_1_Bit_Multiplexer1/2
  2_to_1_Bit_Multiplexer2/1 -> Bit_1/1
  2_to_1_Bit_Multiplexer3/1 -> Bit_1/3
  Logical Operator8/1 -> 2_to_1_Bit_Multiplexer3/2
  Demux/7 -> Logical Operator8/1, 2_to_1_Bit_Multiplexer2/2
  2_to_1_Bit_Multiplexer4/1 -> Bit_2/1
  2_to_1_Bit_Multiplexer5/1 -> Bit_2/3
  Demux/6 -> Logical Operator9/1, 2_to_1_Bit_Multiplexer4/2
  Logical Operator9/1 -> 2_to_1_Bit_Multiplexer5/2
  2_to_1_Bit_Multiplexer7/1 -> Bit_3/3
  2_to_1_Bit_Multiplexer6/1 -> Bit_3/1
  Logical Operator5/1 -> 2_to_1_Bit_Multiplexer7/2
  Demux/5 -> Logical Operator5/1, 2_to_1_Bit_Multiplexer6/2
  Integer to Bit Converter/1 -> Demux/1
  Bit_0/1 -> Mux1/8, Increment Enabled/2
  Logical Operator4/1 -> Logical Operator13/1, 2_to_1_Bit_Multiplexer7/3, 2_to_1_Bit_Multiplexer6/3
  Bit_4/2 -> Terminator4/1
  Bit_5/2 -> Terminator1/1
  Clock/1 -> Bit_0/2, Bit_1/2, Bit_2/2, Bit_3/2, Bit_4/2, Bit_5/2, Bit_6/2, Bit_7/2
  Bit_6/2 -> Terminator2/1
  Increment Enabled1/1 -> 2_to_1_Bit_Multiplexer11/3, 2_to_1_Bit_Multiplexer10/3, Logical Operator1/1
  Bit_5/1 -> Mux1/3, Logical Operator1/2
  Logical Operator1/1 -> 2_to_1_Bit_Multiplexer13/3, 2_to_1_Bit_Multiplexer12/3, Logical Operator2/1
  Bit_7/2 -> Terminator3/1
  Logical Operator2/1 -> 2_to_1_Bit_Multiplexer15/3, 2_to_1_Bit_Multiplexer14/3
  Bit_6/1 -> Mux1/2, Logical Operator2/2
  Bit_7/1 -> Mux1/1
  2_to_1_Bit_Multiplexer9/1 -> Bit_4/3
  2_to_1_Bit_Multiplexer8/1 -> Bit_4/1
  Set_Direct(1b)/1 -> 2_to_1_Bit_Multiplexer12/1, 2_to_1_Bit_Multiplexer13/1, 2_to_1_Bit_Multiplexer14/1, 2_to_1_Bit_Multiplexer15/1, 2_to_1_Bit_Multiplexer10/1, 2_to_1_Bit_Multiplexer11/1, 2_to_1_Bit_Multiplexer8/1, 2_to_1_Bit_Multiplexer9/1, 2_to_1_Bit_Multiplexer6/1, 2_to_1_Bit_Multiplexer7/1, 2_to_1_Bit_Multiplexer4/1, 2_to_1_Bit_Multiplexer5/1, 2_to_1_Bit_Multiplexer3/1, 2_to_1_Bit_Multiplexer2/1, 2_to_1_Bit_Multiplexer/1, 2_to_1_Bit_Multiplexer1/1
  2_to_1_Bit_Multiplexer10/1 -> Bit_5/1
  2_to_1_Bit_Multiplexer11/1 -> Bit_5/3
  Logical Operator10/1 -> 2_to_1_Bit_Multiplexer11/2
  Demux/3 -> Logical Operator10/1, 2_to_1_Bit_Multiplexer10/2
  2_to_1_Bit_Multiplexer12/1 -> Bit_6/1
  2_to_1_Bit_Multiplexer13/1 -> Bit_6/3
  Demux/2 -> Logical Operator11/1, 2_to_1_Bit_Multiplexer12/2
  Logical Operator11/1 -> 2_to_1_Bit_Multiplexer13/2
  2_to_1_Bit_Multiplexer15/1 -> Bit_7/3
  2_to_1_Bit_Multiplexer14/1 -> Bit_7/1
  Logical Operator7/1 -> 2_to_1_Bit_Multiplexer15/2
  Demux/1 -> Logical Operator7/1, 2_to_1_Bit_Multiplexer14/2
  Bit_4/1 -> Mux1/4, Increment Enabled1/2
  Logical Operator12/1 -> 2_to_1_Bit_Multiplexer9/2
  Demux/4 -> Logical Operator12/1, 2_to_1_Bit_Multiplexer8/2
  Logical Operator13/1 -> 2_to_1_Bit_Multiplexer9/3, 2_to_1_Bit_Multiplexer8/3, Increment Enabled1/1

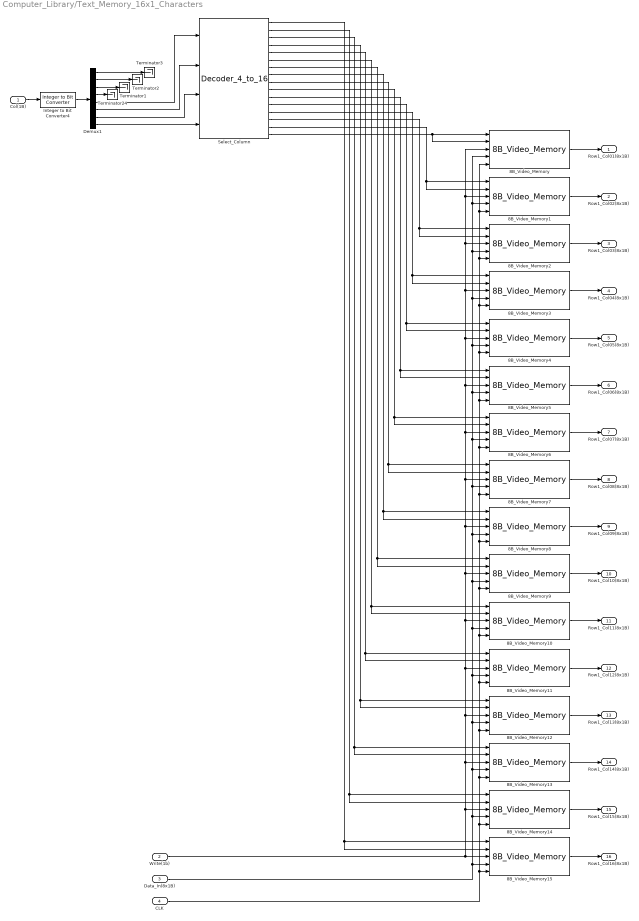
== system Computer_Library/Text_Memory_16x1_Characters ==
  Col(1B) : Inport
  Write(1b) : Inport  Port=2
  Data_In(8x1B) : Inport  Port=3
  CLK : Inport  Port=4
  8B_Video_Memory{,1..15} (16 alike) : Memory_Blocks_Lib/Memory_Blocks_Lib/8B_Video_Memory
  Demux1 : Demux  Outputs=8
  Integer to Bit Converter4 : commutil2/Integer to Bit Converter  nbits=8  signedInputValues=Unsigned  bitOrder=MSB first  outDtype=uint8
  Select_Column : Decoders_Lib/Decoders_Lib/Decoder_4_to_16
  Terminator{1..3,24} (4 alike) : Terminator
  Row1_Col01(8x1B) : Outport
  Row1_Col02(8x1B) : Outport  Port=2
  Row1_Col03(8x1B) : Outport  Port=3
  Row1_Col04(8x1B) : Outport  Port=4
  Row1_Col05(8x1B) : Outport  Port=5
  Row1_Col06(8x1B) : Outport  Port=6
  Row1_Col07(8x1B) : Outport  Port=7
  Row1_Col08(8x1B) : Outport  Port=8
  Row1_Col09(8x1B) : Outport  Port=9
  Row1_Col10(8x1B) : Outport  Port=10
  Row1_Col11(8x1B) : Outport  Port=11
  Row1_Col12(8x1B) : Outport  Port=12
  Row1_Col13(8x1B) : Outport  Port=13
  Row1_Col14(8x1B) : Outport  Port=14
  Row1_Col15(8x1B) : Outport  Port=15
  Row1_Col16(8x1B) : Outport  Port=16
  wires:
  Col(1B)/1 -> Integer to Bit Converter4/1
  Integer to Bit Converter4/1 -> Demux1/1
  Data_In(8x1B)/1 -> 8B_Video_Memory6/4, 8B_Video_Memory5/4, 8B_Video_Memory4/4, 8B_Video_Memory3/4, 8B_Video_Memory2/4, 8B_Video_Memory/4, 8B_Video_Memory1/4, 8B_Video_Memory7/4, 8B_Video_Memory8/4, 8B_Video_Memory9/4, 8B_Video_Memory10/4, 8B_Video_Memory11/4, 8B_Video_Memory12/4, 8B_Video_Memory13/4, 8B_Video_Memory14/4, 8B_Video_Memory15/4
  8B_Video_Memory/1 -> Row1_Col01(8x1B)/1
  8B_Video_Memory1/1 -> Row1_Col02(8x1B)/1
  8B_Video_Memory2/1 -> Row1_Col03(8x1B)/1
  8B_Video_Memory3/1 -> Row1_Col04(8x1B)/1
  CLK/1 -> 8B_Video_Memory6/5, 8B_Video_Memory5/5, 8B_Video_Memory4/5, 8B_Video_Memory3/5, 8B_Video_Memory2/5, 8B_Video_Memory/5, 8B_Video_Memory1/5, 8B_Video_Memory7/5, 8B_Video_Memory8/5, 8B_Video_Memory9/5, 8B_Video_Memory10/5, 8B_Video_Memory11/5, 8B_Video_Memory12/5, 8B_Video_Memory13/5, 8B_Video_Memory14/5, 8B_Video_Memory15/5
  8B_Video_Memory4/1 -> Row1_Col05(8x1B)/1
  8B_Video_Memory5/1 -> Row1_Col06(8x1B)/1
  8B_Video_Memory6/1 -> Row1_Col07(8x1B)/1
  8B_Video_Memory7/1 -> Row1_Col08(8x1B)/1
  8B_Video_Memory8/1 -> Row1_Col09(8x1B)/1
  8B_Video_Memory9/1 -> Row1_Col10(8x1B)/1
  8B_Video_Memory10/1 -> Row1_Col11(8x1B)/1
  8B_Video_Memory11/1 -> Row1_Col12(8x1B)/1
  8B_Video_Memory12/1 -> Row1_Col13(8x1B)/1
  8B_Video_Memory13/1 -> Row1_Col14(8x1B)/1
  8B_Video_Memory14/1 -> Row1_Col15(8x1B)/1
  8B_Video_Memory15/1 -> Row1_Col16(8x1B)/1
  Demux1/5 -> Select_Column/1
  Demux1/6 -> Select_Column/2
  Demux1/8 -> Select_Column/4
  Demux1/7 -> Select_Column/3
  Select_Column/16 -> 8B_Video_Memory/2, 8B_Video_Memory/1
  Select_Column/15 -> 8B_Video_Memory1/2, 8B_Video_Memory1/1
  Write(1b)/1 -> 8B_Video_Memory/3, 8B_Video_Memory1/3, 8B_Video_Memory2/3, 8B_Video_Memory3/3, 8B_Video_Memory4/3, 8B_Video_Memory5/3, 8B_Video_Memory6/3, 8B_Video_Memory7/3, 8B_Video_Memory8/3, 8B_Video_Memory9/3, 8B_Video_Memory10/3, 8B_Video_Memory11/3, 8B_Video_Memory12/3, 8B_Video_Memory13/3, 8B_Video_Memory14/3, 8B_Video_Memory15/3
  Select_Column/14 -> 8B_Video_Memory2/2, 8B_Video_Memory2/1
  Select_Column/13 -> 8B_Video_Memory3/1, 8B_Video_Memory3/2
  Select_Column/12 -> 8B_Video_Memory4/1, 8B_Video_Memory4/2
  Select_Column/11 -> 8B_Video_Memory5/1, 8B_Video_Memory5/2
  Select_Column/10 -> 8B_Video_Memory6/1, 8B_Video_Memory6/2
  Select_Column/9 -> 8B_Video_Memory7/1, 8B_Video_Memory7/2
  Select_Column/8 -> 8B_Video_Memory8/1, 8B_Video_Memory8/2
  Select_Column/7 -> 8B_Video_Memory9/1, 8B_Video_Memory9/2
  Select_Column/6 -> 8B_Video_Memory10/1, 8B_Video_Memory10/2
  Select_Column/5 -> 8B_Video_Memory11/1, 8B_Video_Memory11/2
  Select_Column/4 -> 8B_Video_Memory12/1, 8B_Video_Memory12/2
  Select_Column/3 -> 8B_Video_Memory13/1, 8B_Video_Memory13/2
  Select_Column/2 -> 8B_Video_Memory14/1, 8B_Video_Memory14/2
  Select_Column/1 -> 8B_Video_Memory15/1, 8B_Video_Memory15/2
  Demux1/4 -> Terminator24/1
  Demux1/3 -> Terminator1/1
  Demux1/2 -> Terminator2/1
  Demux1/1 -> Terminator3/1

== system Computer_Library/Text_Memory_2x2_Characters ==
  Row(1B) : Inport
  Col(1B) : Inport  Port=2
  Write(1b) : Inport  Port=3
  Data_In(8x1B) : Inport  Port=4
  CLK : Inport  Port=5
  8B_Video_Memory{,1..3} (4 alike) : Memory_Blocks_Lib/Memory_Blocks_Lib/8B_Video_Memory
  Constant8 : Constant  Value=0  OutDataTypeStr=uint8
  Constant9 : Constant  Value=0  OutDataTypeStr=uint8
  Integer to Bit Converter3 : commutil2/Integer to Bit Converter  nbits=1  signedInputValues=Unsigned  bitOrder=MSB first  outDtype=uint8
  Integer to Bit Converter4 : commutil2/Integer to Bit Converter  nbits=1  signedInputValues=Unsigned  bitOrder=MSB first  outDtype=uint8
  Select_Column : Decoders_Lib/Decoders_Lib/Decoder_2_to_4
  Select_Row : Decoders_Lib/Decoders_Lib/Decoder_2_to_4
  Terminator{1..2,4..5} (4 alike) : Terminator
  Row1_Col1(8x1B) : Outport
  Row1_Col2(8x1B) : Outport  Port=2
  Row2_Col1(8x1B) : Outport  Port=3
  Row2_Col2(8x1B) : Outport  Port=4
  wires:
  Row(1B)/1 -> Integer to Bit Converter3/1
  Integer to Bit Converter3/1 -> Select_Row/2
  Constant8/1 -> Select_Row/1
  Constant9/1 -> Select_Column/1
  Col(1B)/1 -> Integer to Bit Converter4/1
  Integer to Bit Converter4/1 -> Select_Column/2
  Data_In(8x1B)/1 -> 8B_Video_Memory/4, 8B_Video_Memory1/4, 8B_Video_Memory2/4, 8B_Video_Memory3/4
  8B_Video_Memory/1 -> Row1_Col1(8x1B)/1
  8B_Video_Memory1/1 -> Row1_Col2(8x1B)/1
  8B_Video_Memory2/1 -> Row2_Col1(8x1B)/1
  8B_Video_Memory3/1 -> Row2_Col2(8x1B)/1
  CLK/1 -> 8B_Video_Memory/5, 8B_Video_Memory1/5, 8B_Video_Memory2/5, 8B_Video_Memory3/5
  Select_Row/1 -> Terminator4/1
  Select_Row/2 -> Terminator5/1
  Select_Column/1 -> Terminator1/1
  Select_Column/2 -> Terminator2/1
  Select_Row/4 -> 8B_Video_Memory1/2, 8B_Video_Memory/2
  Select_Row/3 -> 8B_Video_Memory3/2, 8B_Video_Memory2/2
  Select_Column/4 -> 8B_Video_Memory2/1, 8B_Video_Memory/1
  Select_Column/3 -> 8B_Video_Memory3/1, 8B_Video_Memory1/1
  Write(1b)/1 -> 8B_Video_Memory/3, 8B_Video_Memory1/3, 8B_Video_Memory2/3, 8B_Video_Memory3/3

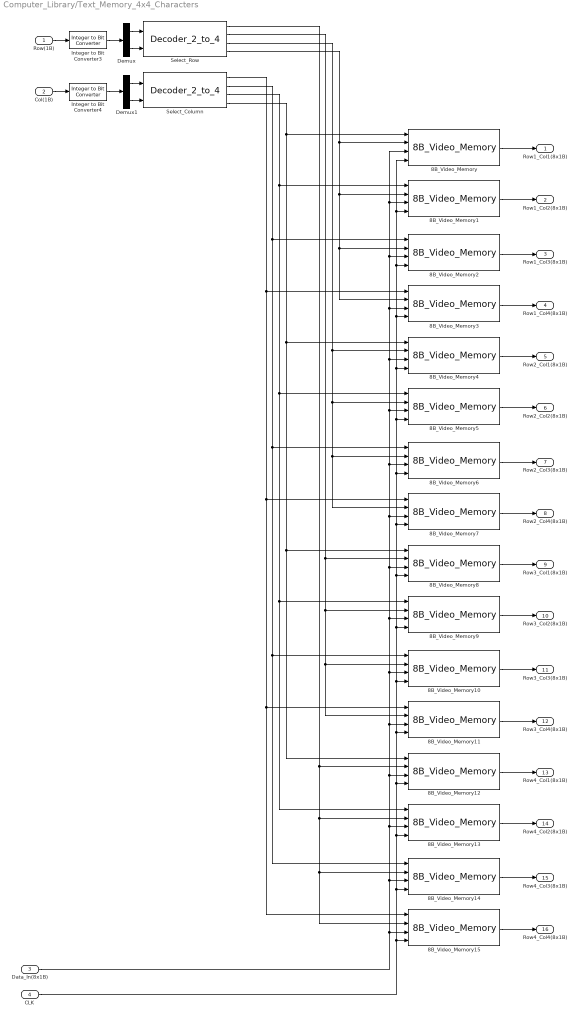
== system Computer_Library/Text_Memory_4x4_Characters ==
  Row(1B) : Inport
  Col(1B) : Inport  Port=2
  Data_In(8x1B) : Inport  Port=3
  CLK : Inport  Port=4
  8B_Video_Memory{,1..15} (16 alike) : Memory_Blocks_Lib/Memory_Blocks_Lib/8B_Video_Memory
  Demux : Demux  Outputs=2
  Demux1 : Demux  Outputs=2
  Integer to Bit Converter3 : commutil2/Integer to Bit Converter  nbits=2  signedInputValues=Unsigned  bitOrder=MSB first  outDtype=uint8
  Integer to Bit Converter4 : commutil2/Integer to Bit Converter  nbits=2  signedInputValues=Unsigned  bitOrder=MSB first  outDtype=uint8
  Select_Column : Decoders_Lib/Decoders_Lib/Decoder_2_to_4
  Select_Row : Decoders_Lib/Decoders_Lib/Decoder_2_to_4
  Row1_Col1(8x1B) : Outport
  Row1_Col2(8x1B) : Outport  Port=2
  Row1_Col3(8x1B) : Outport  Port=3
  Row1_Col4(8x1B) : Outport  Port=4
  Row2_Col1(8x1B) : Outport  Port=5
  Row2_Col2(8x1B) : Outport  Port=6
  Row2_Col3(8x1B) : Outport  Port=7
  Row2_Col4(8x1B) : Outport  Port=8
  Row3_Col1(8x1B) : Outport  Port=9
  Row3_Col2(8x1B) : Outport  Port=10
  Row3_Col3(8x1B) : Outport  Port=11
  Row3_Col4(8x1B) : Outport  Port=12
  Row4_Col1(8x1B) : Outport  Port=13
  Row4_Col2(8x1B) : Outport  Port=14
  Row4_Col3(8x1B) : Outport  Port=15
  Row4_Col4(8x1B) : Outport  Port=16
  wires:
  Row(1B)/1 -> Integer to Bit Converter3/1
  Integer to Bit Converter3/1 -> Demux/1
  Col(1B)/1 -> Integer to Bit Converter4/1
  Integer to Bit Converter4/1 -> Demux1/1
  Data_In(8x1B)/1 -> 8B_Video_Memory15/3, 8B_Video_Memory14/3, 8B_Video_Memory13/3, 8B_Video_Memory12/3, 8B_Video_Memory11/3, 8B_Video_Memory10/3, 8B_Video_Memory9/3, 8B_Video_Memory8/3, 8B_Video_Memory6/3, 8B_Video_Memory5/3, 8B_Video_Memory4/3, 8B_Video_Memory2/3, 8B_Video_Memory1/3, 8B_Video_Memory/3, 8B_Video_Memory3/3, 8B_Video_Memory7/3
  8B_Video_Memory/1 -> Row1_Col1(8x1B)/1
  8B_Video_Memory1/1 -> Row1_Col2(8x1B)/1
  8B_Video_Memory2/1 -> Row1_Col3(8x1B)/1
  8B_Video_Memory3/1 -> Row1_Col4(8x1B)/1
  CLK/1 -> 8B_Video_Memory15/4, 8B_Video_Memory14/4, 8B_Video_Memory13/4, 8B_Video_Memory12/4, 8B_Video_Memory11/4, 8B_Video_Memory10/4, 8B_Video_Memory9/4, 8B_Video_Memory8/4, 8B_Video_Memory7/4, 8B_Video_Memory6/4, 8B_Video_Memory5/4, 8B_Video_Memory4/4, 8B_Video_Memory3/4, 8B_Video_Memory2/4, 8B_Video_Memory1/4, 8B_Video_Memory/4
  Select_Row/1 -> 8B_Video_Memory12/2, 8B_Video_Memory13/2, 8B_Video_Memory14/2, 8B_Video_Memory15/2
  Select_Row/2 -> 8B_Video_Memory8/2, 8B_Video_Memory9/2, 8B_Video_Memory10/2, 8B_Video_Memory11/2
  Select_Column/1 -> 8B_Video_Memory15/1, 8B_Video_Memory11/1, 8B_Video_Memory7/1, 8B_Video_Memory3/1
  Select_Column/2 -> 8B_Video_Memory14/1, 8B_Video_Memory10/1, 8B_Video_Memory6/1, 8B_Video_Memory2/1
  Select_Row/4 -> 8B_Video_Memory/2, 8B_Video_Memory1/2, 8B_Video_Memory2/2, 8B_Video_Memory3/2
  Select_Row/3 -> 8B_Video_Memory4/2, 8B_Video_Memory5/2, 8B_Video_Memory6/2, 8B_Video_Memory7/2
  Select_Column/4 -> 8B_Video_Memory12/1, 8B_Video_Memory8/1, 8B_Video_Memory4/1, 8B_Video_Memory/1
  Select_Column/3 -> 8B_Video_Memory13/1, 8B_Video_Memory9/1, 8B_Video_Memory5/1, 8B_Video_Memory1/1
  8B_Video_Memory4/1 -> Row2_Col1(8x1B)/1
  8B_Video_Memory5/1 -> Row2_Col2(8x1B)/1
  8B_Video_Memory6/1 -> Row2_Col3(8x1B)/1
  8B_Video_Memory7/1 -> Row2_Col4(8x1B)/1
  8B_Video_Memory8/1 -> Row3_Col1(8x1B)/1
  8B_Video_Memory9/1 -> Row3_Col2(8x1B)/1
  8B_Video_Memory10/1 -> Row3_Col3(8x1B)/1
  8B_Video_Memory11/1 -> Row3_Col4(8x1B)/1
  8B_Video_Memory12/1 -> Row4_Col1(8x1B)/1
  8B_Video_Memory13/1 -> Row4_Col2(8x1B)/1
  8B_Video_Memory14/1 -> Row4_Col3(8x1B)/1
  8B_Video_Memory15/1 -> Row4_Col4(8x1B)/1
  Demux/1 -> Select_Row/1
  Demux/2 -> Select_Row/2
  Demux1/1 -> Select_Column/1
  Demux1/2 -> Select_Column/2
